simulink library "csu_mems_mcu_signal_interface_lib"  (R2014b)
settings: Solver=ode45  StartTime=0.0  StopTime=10.0  RelTol=1e-3
libraries: util_info_lib x1
settings Model: Creator=escrane  LastModifiedBy=mstewart

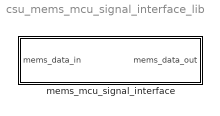
== system csu_mems_mcu_signal_interface_lib ==
  mems_mcu_signal_interface : Subsystem

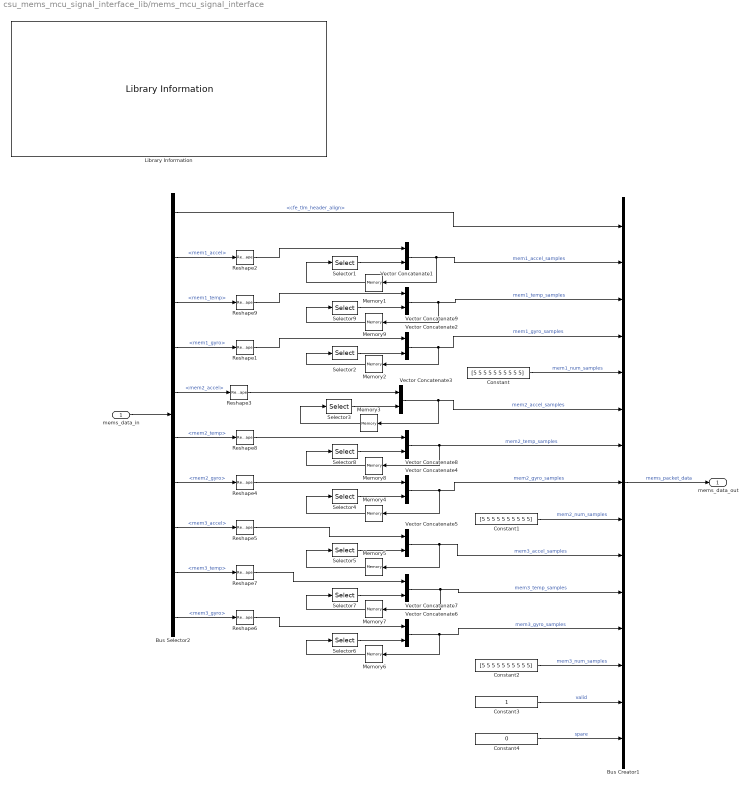
== system csu_mems_mcu_signal_interface_lib/mems_mcu_signal_interface ==
  mems_data_in : Inport
  Bus Selector2 : BusSelector  OutputSignals=cfe_tlm_header_align,mem1_accel,mem1_temp,mem1_gyro,mem2_accel,mem2_temp,mem2_gyro,mem3_accel,mem3_temp,mem3_gyro
  Bus Creator1 : BusCreator  Inputs=15
  Constant : Constant  Value=[5 5 5 5 5 5 5 5 5 5]  OutDataTypeStr=uint8
  Constant1 : Constant  Value=[5 5 5 5 5 5 5 5 5 5]  OutDataTypeStr=uint8
  Constant2 : Constant  Value=[5 5 5 5 5 5 5 5 5 5]  OutDataTypeStr=uint8
  Constant3 : Constant  OutDataTypeStr=uint8
  Constant4 : Constant  Value=0  OutDataTypeStr=uint8
  Library Information : util_info_lib/Library Information  owner='NONE'
  Memory{1..6} (6 alike) : Memory  X0=zeros(10,3)  InheritSampleTime=on
  Memory7 : Memory  X0=zeros(10,1)  InheritSampleTime=on
  Memory8 : Memory  X0=zeros(10,1)  InheritSampleTime=on
  Memory9 : Memory  X0=zeros(10,1)  InheritSampleTime=on
  Reshape{1..6} (6 alike) : Reshape  OutputDimensionality=Row vector (2-D)
  Reshape7 : Reshape  OutputDimensionality=Column vector (2-D)
  Reshape8 : Reshape  OutputDimensionality=Column vector (2-D)
  Reshape9 : Reshape  OutputDimensionality=Column vector (2-D)
  Selector{1..6} (6 alike) : Selector  NumberOfDimensions=2  InputPortWidth=10  IndexOptions=Index vector (dialog),Select all  Indices=[1:9],1  OutputSizes=1,1
  Selector7 : Selector  InputPortWidth=10  Indices=[1:9]
  Selector8 : Selector  InputPortWidth=10  Indices=[1:9]
  Selector9 : Selector  InputPortWidth=10  Indices=[1:9]
  Vector Concatenate{1..9} (9 alike) : Concatenate  Mode=Multidimensional array
  mems_data_out : Outport
  wires:
  Constant4/1 -> Bus Creator1/15  "spare"
  Constant3/1 -> Bus Creator1/14  "valid"
  Constant2/1 -> Bus Creator1/13  "mem3_num_samples"
  Constant1/1 -> Bus Creator1/9  "mem2_num_samples"
  Constant/1 -> Bus Creator1/5  "mem1_num_samples"
  Reshape9/1 -> Vector Concatenate9/1
  Vector Concatenate9/1 -> Memory9/1, Bus Creator1/3  "mem1_temp_samples"
  Selector9/1 -> Vector Concatenate9/2
  Memory9/1 -> Selector9/1
  Bus Selector2/3 -> Reshape9/1  "<mem1_temp>"
  Reshape8/1 -> Vector Concatenate8/1
  Vector Concatenate8/1 -> Bus Creator1/7, Memory8/1  "mem2_temp_samples"
  Selector8/1 -> Vector Concatenate8/2
  Memory8/1 -> Selector8/1
  Bus Selector2/6 -> Reshape8/1  "<mem2_temp>"
  Reshape7/1 -> Vector Concatenate7/1
  Vector Concatenate7/1 -> Bus Creator1/11, Memory7/1  "mem3_temp_samples"
  Selector7/1 -> Vector Concatenate7/2
  Memory7/1 -> Selector7/1
  Bus Selector2/9 -> Reshape7/1  "<mem3_temp>"
  Reshape2/1 -> Vector Concatenate1/1
  Vector Concatenate1/1 -> Bus Creator1/2, Memory1/1  "mem1_accel_samples"
  Selector1/1 -> Vector Concatenate1/2
  Memory1/1 -> Selector1/1
  mems_data_in/1 -> Bus Selector2/1
  Bus Selector2/2 -> Reshape2/1  "<mem1_accel>"
  Bus Creator1/1 -> mems_data_out/1  "mems_packet_data"
  Bus Selector2/1 -> Bus Creator1/1  "<cfe_tlm_header_align>"
  Reshape1/1 -> Vector Concatenate2/1
  Vector Concatenate2/1 -> Memory2/1, Bus Creator1/4  "mem1_gyro_samples"
  Selector2/1 -> Vector Concatenate2/2
  Memory2/1 -> Selector2/1
  Reshape3/1 -> Vector Concatenate3/1
  Vector Concatenate3/1 -> Bus Creator1/6, Memory3/1  "mem2_accel_samples"
  Selector3/1 -> Vector Concatenate3/2
  Memory3/1 -> Selector3/1
  Reshape4/1 -> Vector Concatenate4/1
  Vector Concatenate4/1 -> Memory4/1, Bus Creator1/8  "mem2_gyro_samples"
  Selector4/1 -> Vector Concatenate4/2
  Memory4/1 -> Selector4/1
  Reshape5/1 -> Vector Concatenate5/1
  Vector Concatenate5/1 -> Bus Creator1/10, Memory5/1  "mem3_accel_samples"
  Selector5/1 -> Vector Concatenate5/2
  Memory5/1 -> Selector5/1
  Reshape6/1 -> Vector Concatenate6/1
  Vector Concatenate6/1 -> Bus Creator1/12, Memory6/1  "mem3_gyro_samples"
  Selector6/1 -> Vector Concatenate6/2
  Memory6/1 -> Selector6/1
  Bus Selector2/4 -> Reshape1/1  "<mem1_gyro>"
  Bus Selector2/5 -> Reshape3/1  "<mem2_accel>"
  Bus Selector2/7 -> Reshape4/1  "<mem2_gyro>"
  Bus Selector2/8 -> Reshape5/1  "<mem3_accel>"
  Bus Selector2/10 -> Reshape6/1  "<mem3_gyro>"
